simulink model "dynamicPressure_ul"  (R2018b)
settings: Solver=VariableStepAuto  StartTime=0.0  StopTime=10.0  RelTol=1e-3
settings Model: Creator=mcobb  LastModifiedBy=mcobb

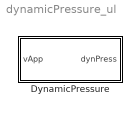
== system dynamicPressure_ul ==
  DynamicPressure : Subsystem  mask{rho=0}
      mask prompts: rho "Fluid density"

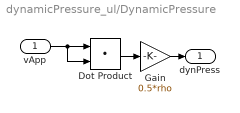
== system dynamicPressure_ul/DynamicPressure ==
  vApp : Inport
  Dot Product : DotProduct  InputSameDT=on  OutDataTypeStr=Inherit: Inherit via internal rule
  Gain : Gain  Gain=0.5*rho
  dynPress : Outport
  wires:
  Gain/1 -> dynPress/1
  vApp/1 -> Dot Product/2, Dot Product/1
  Dot Product/1 -> Gain/1
